simulink model "simulation_Hippocampus_compare_paper"  (R2023a)
settings: Solver=ode3  StartTime=0  StopTime=120  FixedStep=0.001  MaxStep=0.001  MinStep=0.00001  RelTol=1e-5  AbsTol=1e-5  EnableMultiTasking=on
values from neighbouring files (symbols this model uses):
  k_pos_ndi = 8    [parameters.m]
  k_vel_ndi = 8    [parameters.m]
  Kf = 6    [parameters.m]
  Kp = 0.01    [parameters.m]
  Kp_p = 30    [parameters.m]
  Kp_pitch = 8    [parameters.m]
  Kp_q = 10    [parameters.m]
  Kp_r = 10    [parameters.m]
  Kp_roll = 10    [parameters.m]
  Kp_u = 8    [parameters.m]
  Kp_yaw = 8    [parameters.m]
  Kq = 5    [parameters.m]
  Kr = 8    [parameters.m]
  Ktau1 = 0.1    [parameters.m]
  Ktau2 = 5    [parameters.m]
  Ktau3 = 5    [parameters.m]
  Ku = 8    [parameters.m]
  p11 = 0.4    [parameters.m]
  p12 = 0.2    [parameters.m]
  p21 = 0.2    [parameters.m]
  p22 = 0.05    [parameters.m]
  p31 = 0.3    [parameters.m]
  p32 = 0.05    [parameters.m]
  p41 = 0.5    [parameters.m]
  p42 = 0.1    [parameters.m]
  p51 = 0.5    [parameters.m]
  p52 = 0.1    [parameters.m]
  p61 = 0.5    [parameters.m]
  p62 = 0.1    [parameters.m]
  Q1 = -8    [simulation_para.m]
  Q2 = -10    [simulation_para.m]
  Q3 = -[0.01,5,8]    [simulation_para.m]
  Q4 = -[0.001,0.1,0.1]    [simulation_para.m]
  r1 = 4    [parameters.m]
  r2 = 6    [parameters.m]
libraries: simulink x8
(part 3 of 7)

== system simulation_Hippocampus_compare_paper/Proposed Linear gain/Disturbance: All derivatives2/disturbance3 ==
  note: Subsystem
  a : Inport
  a1 : Inport  Port=2
  Constant : Constant  Value=10
  Constant2 : Constant  Value=10
  Constant3 : Constant  Value=45
  Constant4 : Constant  Value=20
  Gain : Gain  Gain=pi/180
  Gain1 : Gain  Gain=pi/180
  MATLAB Function : MATLAB Function  TreatAsAtomicUnit=on
  Mux : Mux  Inputs=3
  Subsystem1 : Subsystem
  d : Outport
  wires:
  Subsystem1/1(Out1) -> MATLAB Function/3(u_wave)
  Constant/1 -> MATLAB Function/5(u_un)
  Mux/1 -> MATLAB Function/4(u_c)
  MATLAB Function/1(d) -> d/1
  a1/1 -> MATLAB Function/1(p)
  a/1 -> MATLAB Function/2(a)
  Constant4/1 -> Mux/1
  Gain/1 -> Mux/2
  Gain1/1 -> Mux/3
  Constant3/1 -> Gain1/1
  Constant2/1 -> Gain/1

== system simulation_Hippocampus_compare_paper/Proposed Linear gain/Disturbance: All derivatives2/old disturbance ==
  Gain : Gain  Gain=ones(12,1)  Multiplication=Matrix(K*u)
  Step : Step  Time=50  After=0.5  SampleTime=0
  Step1 : Step  Time=55  After=-0.5  SampleTime=0
  Step2 : Step  Time=100  After=0.5  SampleTime=0
  Step3 : Step  Time=105  After=-0.5  SampleTime=0
  Sum : Sum  Inputs=|++
  Sum2 : Sum  Inputs=|++
  Sum3 : Sum  Inputs=|++
  Out1 : Outport
  wires:
  Gain/1 -> Out1/1
  Sum3/1 -> Gain/1
  Step3/1 -> Sum2/2
  Step/1 -> Sum/1
  Step1/1 -> Sum/2
  Step2/1 -> Sum2/1
  Sum/1 -> Sum3/1
  Sum2/1 -> Sum3/2

== system simulation_Hippocampus_compare_paper/Proposed Linear gain/HippCampus/Subsystem ==
  In1 : Inport
  Demux : Demux  Outputs=[5 1 1 1 4]
  MATLAB Function : MATLAB Function  TreatAsAtomicUnit=on
  Mux : Mux  Inputs=5
  state : Outport
  wires:
  Demux/2 -> MATLAB Function/1(u)
  MATLAB Function/1(y) -> Mux/2
  In1/1 -> Demux/1
  Demux/3 -> Mux/3
  Demux/1 -> Mux/1
  Mux/1 -> state/1
  Demux/5 -> Mux/5
  Demux/4 -> Mux/4

== system simulation_Hippocampus_compare_paper/Proposed Linear gain/HippCampus/Subsystem1 ==
  u : Inport
  Integrator2 : Integrator
  Sqrt1 : Sqrt
  norm1 : MATLAB Function  TreatAsAtomicUnit=on
  Out1 : Outport
  wires:
  norm1/1(y) -> Integrator2/1
  Sqrt1/1 -> Out1/1
  Integrator2/1 -> Sqrt1/1
  u/1 -> norm1/1(u)

== system simulation_Hippocampus_compare_paper/Proposed Linear gain/HippCampus/Subsystem4 ==
  u : Inport
  Demux : Demux
  Mux : Mux
  Subsystem : Subsystem
  Subsystem1 : Subsystem
  Subsystem2 : Subsystem
  Subsystem3 : Subsystem
  Out1 : Outport
  wires:
  Subsystem2/1(Out1) -> Mux/3
  Demux/4 -> Subsystem3/1(u)
  Demux/3 -> Subsystem2/1(u)
  Subsystem1/1(Out1) -> Mux/2
  Demux/2 -> Subsystem1/1(u)
  Subsystem3/1(Out1) -> Mux/4
  Demux/1 -> Subsystem/1(u)
  Subsystem/1(Out1) -> Mux/1
  Mux/1 -> Out1/1
  u/1 -> Demux/1

== system simulation_Hippocampus_compare_paper/Proposed Linear gain1/Controller/calculate derivative 1 ==
  In1 : Inport
  Clock : Clock
  Derivative : Derivative
  MATLAB Function : MATLAB Function  TreatAsAtomicUnit=on
  Saturation : Saturate  UpperLimit=[6;3;6;6]  LowerLimit=-[6;3;6;6]
  y : Outport
  wires:
  Clock/1 -> MATLAB Function/2(t)
  In1/1 -> Derivative/1
  MATLAB Function/1(y) -> Saturation/1
  Derivative/1 -> MATLAB Function/1(u)
  Saturation/1 -> y/1

== system simulation_Hippocampus_compare_paper/Proposed Linear gain1/Disturbance: All derivatives1/disturbance2 ==
  Gain : Gain  Gain=[0;0;0;0;0;0;1;1;1;1;1;1]  Multiplication=Matrix(K*u)
  Step2 : Step  Time=60  After=0.5  SampleTime=0
  Step3 : Step  Time=55  After=0  SampleTime=0
  Sum1 : Sum
  Out1 : Outport
  wires:
  Step2/1 -> Sum1/1
  Step3/1 -> Sum1/2
  Gain/1 -> Out1/1
  Sum1/1 -> Gain/1

== system simulation_Hippocampus_compare_paper/Proposed Linear gain1/Disturbance: All derivatives1/disturbance3 ==
  note: Subsystem
  a : Inport
  a1 : Inport  Port=2
  Constant : Constant  Value=10
  Constant2 : Constant  Value=10
  Constant3 : Constant  Value=45
  Constant4 : Constant  Value=20
  Gain : Gain  Gain=pi/180
  Gain1 : Gain  Gain=pi/180
  MATLAB Function : MATLAB Function  TreatAsAtomicUnit=on
  Mux : Mux  Inputs=3
  Subsystem1 : Subsystem
  d : Outport
  wires:
  Subsystem1/1(Out1) -> MATLAB Function/3(u_wave)
  Constant/1 -> MATLAB Function/5(u_un)
  Mux/1 -> MATLAB Function/4(u_c)
  MATLAB Function/1(d) -> d/1
  a1/1 -> MATLAB Function/1(p)
  a/1 -> MATLAB Function/2(a)
  Constant4/1 -> Mux/1
  Gain/1 -> Mux/2
  Gain1/1 -> Mux/3
  Constant3/1 -> Gain1/1
  Constant2/1 -> Gain/1

== system simulation_Hippocampus_compare_paper/Proposed Linear gain1/Disturbance: All derivatives1/old disturbance ==
  Gain : Gain  Gain=ones(12,1)  Multiplication=Matrix(K*u)
  Step : Step  Time=50  After=0.5  SampleTime=0
  Step1 : Step  Time=55  After=-0.5  SampleTime=0
  Step2 : Step  Time=100  After=0.5  SampleTime=0
  Step3 : Step  Time=105  After=-0.5  SampleTime=0
  Sum : Sum  Inputs=|++
  Sum2 : Sum  Inputs=|++
  Sum3 : Sum  Inputs=|++
  Out1 : Outport
  wires:
  Gain/1 -> Out1/1
  Sum3/1 -> Gain/1
  Step3/1 -> Sum2/2
  Step/1 -> Sum/1
  Step1/1 -> Sum/2
  Step2/1 -> Sum2/1
  Sum/1 -> Sum3/1
  Sum2/1 -> Sum3/2

== system simulation_Hippocampus_compare_paper/Proposed Linear gain1/HippCampus/Subsystem ==
  In1 : Inport
  Demux : Demux  Outputs=[5 1 1 1 4]
  MATLAB Function : MATLAB Function  TreatAsAtomicUnit=on
  Mux : Mux  Inputs=5
  state : Outport
  wires:
  Demux/2 -> MATLAB Function/1(u)
  MATLAB Function/1(y) -> Mux/2
  In1/1 -> Demux/1
  Demux/3 -> Mux/3
  Demux/1 -> Mux/1
  Mux/1 -> state/1
  Demux/5 -> Mux/5
  Demux/4 -> Mux/4

== system simulation_Hippocampus_compare_paper/Proposed Linear gain1/HippCampus/Subsystem1 ==
  u : Inport
  Integrator2 : Integrator
  Sqrt1 : Sqrt
  norm1 : MATLAB Function  TreatAsAtomicUnit=on
  Out1 : Outport
  wires:
  norm1/1(y) -> Integrator2/1
  Sqrt1/1 -> Out1/1
  Integrator2/1 -> Sqrt1/1
  u/1 -> norm1/1(u)

== system simulation_Hippocampus_compare_paper/Proposed Linear gain1/HippCampus/Subsystem4 ==
  u : Inport
  Demux : Demux
  Mux : Mux
  Subsystem : Subsystem
  Subsystem1 : Subsystem
  Subsystem2 : Subsystem
  Subsystem3 : Subsystem
  Out1 : Outport
  wires:
  Subsystem2/1(Out1) -> Mux/3
  Demux/4 -> Subsystem3/1(u)
  Demux/3 -> Subsystem2/1(u)
  Subsystem1/1(Out1) -> Mux/2
  Demux/2 -> Subsystem1/1(u)
  Subsystem3/1(Out1) -> Mux/4
  Demux/1 -> Subsystem/1(u)
  Subsystem/1(Out1) -> Mux/1
  Mux/1 -> Out1/1
  u/1 -> Demux/1

== system simulation_Hippocampus_compare_paper/Proposed nonlinear gain/Controller/calculate derivative 1 ==
  In1 : Inport
  Clock : Clock
  Derivative : Derivative
  MATLAB Function : MATLAB Function  TreatAsAtomicUnit=on
  Saturation : Saturate  UpperLimit=[6;3;6;6]  LowerLimit=-[6;3;6;6]
  y : Outport
  wires:
  Clock/1 -> MATLAB Function/2(t)
  In1/1 -> Derivative/1
  MATLAB Function/1(y) -> Saturation/1
  Derivative/1 -> MATLAB Function/1(u)
  Saturation/1 -> y/1

== system simulation_Hippocampus_compare_paper/Proposed nonlinear gain/Disturbance: All derivatives1/disturbance2 ==
  Gain : Gain  Gain=[0;0;0;0;0;0;1;1;1;1;1;1]  Multiplication=Matrix(K*u)
  Step2 : Step  Time=60  After=0.5  SampleTime=0
  Step3 : Step  Time=55  After=0  SampleTime=0
  Sum1 : Sum
  Out1 : Outport
  wires:
  Step2/1 -> Sum1/1
  Step3/1 -> Sum1/2
  Gain/1 -> Out1/1
  Sum1/1 -> Gain/1

== system simulation_Hippocampus_compare_paper/Proposed nonlinear gain/Disturbance: All derivatives1/disturbance3 ==
  note: Subsystem
  a : Inport
  a1 : Inport  Port=2
  Constant : Constant  Value=10
  Constant2 : Constant  Value=10
  Constant3 : Constant  Value=45
  Constant4 : Constant  Value=20
  Gain : Gain  Gain=pi/180
  Gain1 : Gain  Gain=pi/180
  MATLAB Function : MATLAB Function  TreatAsAtomicUnit=on
  Mux : Mux  Inputs=3
  Subsystem1 : Subsystem
  d : Outport
  wires:
  Subsystem1/1(Out1) -> MATLAB Function/3(u_wave)
  Constant/1 -> MATLAB Function/5(u_un)
  Mux/1 -> MATLAB Function/4(u_c)
  MATLAB Function/1(d) -> d/1
  a1/1 -> MATLAB Function/1(p)
  a/1 -> MATLAB Function/2(a)
  Constant4/1 -> Mux/1
  Gain/1 -> Mux/2
  Gain1/1 -> Mux/3
  Constant3/1 -> Gain1/1
  Constant2/1 -> Gain/1

== system simulation_Hippocampus_compare_paper/Proposed nonlinear gain/Disturbance: All derivatives1/old disturbance ==
  Gain : Gain  Gain=ones(12,1)  Multiplication=Matrix(K*u)
  Step : Step  Time=50  After=0.5  SampleTime=0
  Step1 : Step  Time=55  After=-0.5  SampleTime=0
  Step2 : Step  Time=100  After=0.5  SampleTime=0
  Step3 : Step  Time=105  After=-0.5  SampleTime=0
  Sum : Sum  Inputs=|++
  Sum2 : Sum  Inputs=|++
  Sum3 : Sum  Inputs=|++
  Out1 : Outport
  wires:
  Gain/1 -> Out1/1
  Sum3/1 -> Gain/1
  Step3/1 -> Sum2/2
  Step/1 -> Sum/1
  Step1/1 -> Sum/2
  Step2/1 -> Sum2/1
  Sum/1 -> Sum3/1
  Sum2/1 -> Sum3/2

== system simulation_Hippocampus_compare_paper/Proposed nonlinear gain/HippCampus/Subsystem ==
  In1 : Inport
  Demux : Demux  Outputs=[5 1 1 1 4]
  MATLAB Function : MATLAB Function  TreatAsAtomicUnit=on
  Mux : Mux  Inputs=5
  state : Outport
  wires:
  Demux/2 -> MATLAB Function/1(u)
  MATLAB Function/1(y) -> Mux/2
  In1/1 -> Demux/1
  Demux/3 -> Mux/3
  Demux/1 -> Mux/1
  Mux/1 -> state/1
  Demux/5 -> Mux/5
  Demux/4 -> Mux/4

== system simulation_Hippocampus_compare_paper/Proposed nonlinear gain/HippCampus/Subsystem1 ==
  u : Inport
  Integrator2 : Integrator
  Sqrt1 : Sqrt
  norm1 : MATLAB Function  TreatAsAtomicUnit=on
  Out1 : Outport
  wires:
  norm1/1(y) -> Integrator2/1
  Sqrt1/1 -> Out1/1
  Integrator2/1 -> Sqrt1/1
  u/1 -> norm1/1(u)

== system simulation_Hippocampus_compare_paper/Proposed nonlinear gain/HippCampus/Subsystem4 ==
  u : Inport
  Demux : Demux
  Mux : Mux
  Subsystem : Subsystem
  Subsystem1 : Subsystem
  Subsystem2 : Subsystem
  Subsystem3 : Subsystem
  Out1 : Outport
  wires:
  Subsystem2/1(Out1) -> Mux/3
  Demux/4 -> Subsystem3/1(u)
  Demux/3 -> Subsystem2/1(u)
  Subsystem1/1(Out1) -> Mux/2
  Demux/2 -> Subsystem1/1(u)
  Subsystem3/1(Out1) -> Mux/4
  Demux/1 -> Subsystem/1(u)
  Subsystem/1(Out1) -> Mux/1
  Mux/1 -> Out1/1
  u/1 -> Demux/1

== system simulation_Hippocampus_compare_paper/Proposed nonlinear gain1/Controller/calculate derivative 1 ==
  In1 : Inport
  Clock : Clock
  Derivative : Derivative
  MATLAB Function : MATLAB Function  TreatAsAtomicUnit=on
  Saturation : Saturate  UpperLimit=[6;3;6;6]  LowerLimit=-[6;3;6;6]
  y : Outport
  wires:
  Clock/1 -> MATLAB Function/2(t)
  In1/1 -> Derivative/1
  MATLAB Function/1(y) -> Saturation/1
  Derivative/1 -> MATLAB Function/1(u)
  Saturation/1 -> y/1

== system simulation_Hippocampus_compare_paper/Proposed nonlinear gain1/Disturbance: All derivatives1/disturbance2 ==
  Gain : Gain  Gain=[0;0;0;0;0;0;1;1;1;1;1;1]  Multiplication=Matrix(K*u)
  Step2 : Step  Time=60  After=0.5  SampleTime=0
  Step3 : Step  Time=55  After=0  SampleTime=0
  Sum1 : Sum
  Out1 : Outport
  wires:
  Step2/1 -> Sum1/1
  Step3/1 -> Sum1/2
  Gain/1 -> Out1/1
  Sum1/1 -> Gain/1

== system simulation_Hippocampus_compare_paper/Proposed nonlinear gain1/Disturbance: All derivatives1/disturbance3 ==
  note: Subsystem
  a : Inport
  a1 : Inport  Port=2
  Constant : Constant  Value=10
  Constant2 : Constant  Value=10
  Constant3 : Constant  Value=45
  Constant4 : Constant  Value=20
  Gain : Gain  Gain=pi/180
  Gain1 : Gain  Gain=pi/180
  MATLAB Function : MATLAB Function  TreatAsAtomicUnit=on
  Mux : Mux  Inputs=3
  Subsystem1 : Subsystem
  d : Outport
  wires:
  Subsystem1/1(Out1) -> MATLAB Function/3(u_wave)
  Constant/1 -> MATLAB Function/5(u_un)
  Mux/1 -> MATLAB Function/4(u_c)
  MATLAB Function/1(d) -> d/1
  a1/1 -> MATLAB Function/1(p)
  a/1 -> MATLAB Function/2(a)
  Constant4/1 -> Mux/1
  Gain/1 -> Mux/2
  Gain1/1 -> Mux/3
  Constant3/1 -> Gain1/1
  Constant2/1 -> Gain/1

== system simulation_Hippocampus_compare_paper/Proposed nonlinear gain1/Disturbance: All derivatives1/old disturbance ==
  Gain : Gain  Gain=ones(12,1)  Multiplication=Matrix(K*u)
  Step : Step  Time=50  After=0.5  SampleTime=0
  Step1 : Step  Time=55  After=-0.5  SampleTime=0
  Step2 : Step  Time=100  After=0.5  SampleTime=0
  Step3 : Step  Time=105  After=-0.5  SampleTime=0
  Sum : Sum  Inputs=|++
  Sum2 : Sum  Inputs=|++
  Sum3 : Sum  Inputs=|++
  Out1 : Outport
  wires:
  Gain/1 -> Out1/1
  Sum3/1 -> Gain/1
  Step3/1 -> Sum2/2
  Step/1 -> Sum/1
  Step1/1 -> Sum/2
  Step2/1 -> Sum2/1
  Sum/1 -> Sum3/1
  Sum2/1 -> Sum3/2

== system simulation_Hippocampus_compare_paper/Proposed nonlinear gain1/HippCampus/Subsystem ==
  In1 : Inport
  Demux : Demux  Outputs=[5 1 1 1 4]
  MATLAB Function : MATLAB Function  TreatAsAtomicUnit=on
  Mux : Mux  Inputs=5
  state : Outport
  wires:
  Demux/2 -> MATLAB Function/1(u)
  MATLAB Function/1(y) -> Mux/2
  In1/1 -> Demux/1
  Demux/3 -> Mux/3
  Demux/1 -> Mux/1
  Mux/1 -> state/1
  Demux/5 -> Mux/5
  Demux/4 -> Mux/4

== system simulation_Hippocampus_compare_paper/Proposed nonlinear gain1/HippCampus/Subsystem1 ==
  u : Inport
  Integrator2 : Integrator
  Sqrt1 : Sqrt
  norm1 : MATLAB Function  TreatAsAtomicUnit=on
  Out1 : Outport
  wires:
  norm1/1(y) -> Integrator2/1
  Sqrt1/1 -> Out1/1
  Integrator2/1 -> Sqrt1/1
  u/1 -> norm1/1(u)

== system simulation_Hippocampus_compare_paper/Proposed nonlinear gain1/HippCampus/Subsystem4 ==
  u : Inport
  Demux : Demux
  Mux : Mux
  Subsystem : Subsystem
  Subsystem1 : Subsystem
  Subsystem2 : Subsystem
  Subsystem3 : Subsystem
  Out1 : Outport
  wires:
  Subsystem2/1(Out1) -> Mux/3
  Demux/4 -> Subsystem3/1(u)
  Demux/3 -> Subsystem2/1(u)
  Subsystem1/1(Out1) -> Mux/2
  Demux/2 -> Subsystem1/1(u)
  Subsystem3/1(Out1) -> Mux/4
  Demux/1 -> Subsystem/1(u)
  Subsystem/1(Out1) -> Mux/1
  Mux/1 -> Out1/1
  u/1 -> Demux/1

== system simulation_Hippocampus_compare_paper/Proposed nonlinear gain2/Controller/calculate derivative 1 ==
  In1 : Inport
  Clock : Clock
  Derivative : Derivative
  MATLAB Function : MATLAB Function  TreatAsAtomicUnit=on
  Saturation : Saturate  UpperLimit=[6;3;6;6]  LowerLimit=-[6;3;6;6]
  y : Outport
  wires:
  Clock/1 -> MATLAB Function/2(t)
  In1/1 -> Derivative/1
  MATLAB Function/1(y) -> Saturation/1
  Derivative/1 -> MATLAB Function/1(u)
  Saturation/1 -> y/1

== system simulation_Hippocampus_compare_paper/Proposed nonlinear gain2/HippCampus/Subsystem ==
  In1 : Inport
  Demux : Demux  Outputs=[5 1 1 1 4]
  MATLAB Function : MATLAB Function  TreatAsAtomicUnit=on
  Mux : Mux  Inputs=5
  state : Outport
  wires:
  Demux/2 -> MATLAB Function/1(u)
  MATLAB Function/1(y) -> Mux/2
  In1/1 -> Demux/1
  Demux/3 -> Mux/3
  Demux/1 -> Mux/1
  Mux/1 -> state/1
  Demux/5 -> Mux/5
  Demux/4 -> Mux/4

== system simulation_Hippocampus_compare_paper/Proposed nonlinear gain2/HippCampus/Subsystem1 ==
  u : Inport
  Integrator2 : Integrator
  Sqrt1 : Sqrt
  norm1 : MATLAB Function  TreatAsAtomicUnit=on
  Out1 : Outport
  wires:
  norm1/1(y) -> Integrator2/1
  Sqrt1/1 -> Out1/1
  Integrator2/1 -> Sqrt1/1
  u/1 -> norm1/1(u)

== system simulation_Hippocampus_compare_paper/Proposed nonlinear gain2/HippCampus/Subsystem4 ==
  u : Inport
  Demux : Demux
  Mux : Mux
  Subsystem : Subsystem
  Subsystem1 : Subsystem
  Subsystem2 : Subsystem
  Subsystem3 : Subsystem
  Out1 : Outport
  wires:
  Subsystem2/1(Out1) -> Mux/3
  Demux/4 -> Subsystem3/1(u)
  Demux/3 -> Subsystem2/1(u)
  Subsystem1/1(Out1) -> Mux/2
  Demux/2 -> Subsystem1/1(u)
  Subsystem3/1(Out1) -> Mux/4
  Demux/1 -> Subsystem/1(u)
  Subsystem/1(Out1) -> Mux/1
  Mux/1 -> Out1/1
  u/1 -> Demux/1

== system simulation_Hippocampus_compare_paper/Stabilizing without v w /Controller/calculate derivative 1 ==
  In1 : Inport
  Clock : Clock
  Derivative : Derivative
  MATLAB Function : MATLAB Function  TreatAsAtomicUnit=on
  Saturation : Saturate  UpperLimit=[6;3;6;6]  LowerLimit=-[6;3;6;6]
  y : Outport
  wires:
  Clock/1 -> MATLAB Function/2(t)
  In1/1 -> Derivative/1
  MATLAB Function/1(y) -> Saturation/1
  Derivative/1 -> MATLAB Function/1(u)
  Saturation/1 -> y/1

== system simulation_Hippocampus_compare_paper/Stabilizing without v w /HippCampus/Subsystem ==
  In1 : Inport
  Demux : Demux  Outputs=[5 1 1 1 4]
  MATLAB Function : MATLAB Function  TreatAsAtomicUnit=on
  Mux : Mux  Inputs=5
  state : Outport
  wires:
  Demux/2 -> MATLAB Function/1(u)
  MATLAB Function/1(y) -> Mux/2
  In1/1 -> Demux/1
  Demux/3 -> Mux/3
  Demux/1 -> Mux/1
  Mux/1 -> state/1
  Demux/5 -> Mux/5
  Demux/4 -> Mux/4

== system simulation_Hippocampus_compare_paper/Stabilizing without v w /HippCampus/Subsystem1 ==
  u : Inport
  Integrator2 : Integrator
  Sqrt1 : Sqrt
  norm1 : MATLAB Function  TreatAsAtomicUnit=on
  Out1 : Outport
  wires:
  norm1/1(y) -> Integrator2/1
  Sqrt1/1 -> Out1/1
  Integrator2/1 -> Sqrt1/1
  u/1 -> norm1/1(u)

== system simulation_Hippocampus_compare_paper/Stabilizing without v w /HippCampus/Subsystem4 ==
  u : Inport
  Demux : Demux
  Mux : Mux
  Subsystem : Subsystem
  Subsystem1 : Subsystem
  Subsystem2 : Subsystem
  Subsystem3 : Subsystem
  Out1 : Outport
  wires:
  Subsystem2/1(Out1) -> Mux/3
  Demux/4 -> Subsystem3/1(u)
  Demux/3 -> Subsystem2/1(u)
  Subsystem1/1(Out1) -> Mux/2
  Demux/2 -> Subsystem1/1(u)
  Subsystem3/1(Out1) -> Mux/4
  Demux/1 -> Subsystem/1(u)
  Subsystem/1(Out1) -> Mux/1
  Mux/1 -> Out1/1
  u/1 -> Demux/1

== system simulation_Hippocampus_compare_paper/Stabilizing without v w 1/Controller/calculate derivative  ==
  In1 : Inport
  Clock : Clock
  Derivative : Derivative
  MATLAB Function : MATLAB Function  TreatAsAtomicUnit=on
  Saturation : Saturate  UpperLimit=[10;10;10;10]  LowerLimit=-[10;10;10;10]
  y : Outport
  wires:
  Clock/1 -> MATLAB Function/2(t)
  In1/1 -> Derivative/1
  MATLAB Function/1(y) -> Saturation/1
  Derivative/1 -> MATLAB Function/1(u)
  Saturation/1 -> y/1

== system simulation_Hippocampus_compare_paper/Stabilizing without v w 1/HippCampus/Subsystem ==
  In1 : Inport
  Demux : Demux  Outputs=[5 1 1 1 4]
  MATLAB Function : MATLAB Function  TreatAsAtomicUnit=on
  Mux : Mux  Inputs=5
  state : Outport
  wires:
  Demux/2 -> MATLAB Function/1(u)
  MATLAB Function/1(y) -> Mux/2
  In1/1 -> Demux/1
  Demux/3 -> Mux/3
  Demux/1 -> Mux/1
  Mux/1 -> state/1
  Demux/5 -> Mux/5
  Demux/4 -> Mux/4

== system simulation_Hippocampus_compare_paper/Stabilizing without v w 1/HippCampus/Subsystem1 ==
  u : Inport
  Integrator2 : Integrator
  Sqrt1 : Sqrt
  norm1 : MATLAB Function  TreatAsAtomicUnit=on
  Out1 : Outport
  wires:
  norm1/1(y) -> Integrator2/1
  Sqrt1/1 -> Out1/1
  Integrator2/1 -> Sqrt1/1
  u/1 -> norm1/1(u)

== system simulation_Hippocampus_compare_paper/Stabilizing without v w 1/HippCampus/Subsystem4 ==
  u : Inport
  Demux : Demux
  Mux : Mux
  Subsystem : Subsystem
  Subsystem1 : Subsystem
  Subsystem2 : Subsystem
  Subsystem3 : Subsystem
  Out1 : Outport
  wires:
  Subsystem2/1(Out1) -> Mux/3
  Demux/4 -> Subsystem3/1(u)
  Demux/3 -> Subsystem2/1(u)
  Subsystem1/1(Out1) -> Mux/2
  Demux/2 -> Subsystem1/1(u)
  Subsystem3/1(Out1) -> Mux/4
  Demux/1 -> Subsystem/1(u)
  Subsystem/1(Out1) -> Mux/1
  Mux/1 -> Out1/1
  u/1 -> Demux/1

== system simulation_Hippocampus_compare_paper/NDI/Controller/Subsystem/Subsystem1 ==
  rpy_ref : Inport
  state : Inport  Port=2
  Add1 : Sum  Inputs=+-
  Add2 : Sum  Inputs=+-
  Add3 : Sum  Inputs=+-
  Demux1 : Demux  Outputs=3
  Demux2 : Demux  Outputs=3
  Gain : Gain  Gain=Kp_roll
  Gain1 : Gain  Gain=Kp_yaw
  Gain2 : Gain  Gain=Kp_pitch
  Mux2 : Mux  Inputs=3
  Subsystem : Subsystem
  pqr_ref : Outport
  wires:
  state/1 -> Subsystem/1(x)
  Demux1/1 -> Add1/2
  Demux1/3 -> Add3/2
  Demux2/3 -> Add3/1
  Demux1/2 -> Add2/2
  Gain/1 -> Mux2/1
  Gain1/1 -> Mux2/3
  Add2/1 -> Gain2/1
  Gain2/1 -> Mux2/2
  Demux2/2 -> Add2/1
  Demux2/1 -> Add1/1
  Subsystem/1(rpy) -> Demux1/1
  rpy_ref/1 -> Demux2/1
  Add1/1 -> Gain/1
  Add3/1 -> Gain1/1
  Mux2/1 -> pqr_ref/1

== system simulation_Hippocampus_compare_paper/NDI/Controller/Subsystem/Subsystem2 ==
  state : Inport
  upqr_ref : Inport  Port=2
  Add{,1..4} (5 alike) : Sum  Inputs=+-
  Demux : Demux
  Demux1 : Demux
  Divide : Product  Inputs=**  Multiplication=Matrix(*)
  Gain : Gain  Gain=Kp_p
  Gain1 : Gain  Gain=Kp_r
  Gain2 : Gain  Gain=Kp_q
  Gain3 : Gain  Gain=Kp_u
  Mux : Mux
  NDI : Subsystem
  Subsystem : Subsystem
  tau : Outport
  wires:
  Add1/1 -> Gain/1
  NDI/1(Lg_h_inv) -> Divide/1
  Mux/1 -> Add/1
  Add2/1 -> Gain2/1
  Add3/1 -> Gain1/1
  Divide/1 -> tau/1
  NDI/2(Lf_h) -> Add/2
  Add/1 -> Divide/2
  state/1 -> Subsystem/1(x), NDI/1(state)
  Subsystem/1(upqr) -> Demux/1
  Demux1/2 -> Add1/1
  Demux1/3 -> Add2/1
  Demux1/4 -> Add3/1
  upqr_ref/1 -> Demux1/1
  Gain1/1 -> Mux/4
  Gain2/1 -> Mux/3
  Gain/1 -> Mux/2
  Add4/1 -> Gain3/1
  Gain3/1 -> Mux/1
  Demux/1 -> Add4/2
  Demux/2 -> Add1/2
  Demux/3 -> Add2/2
  Demux/4 -> Add3/2
  Demux1/1 -> Add4/1

== system simulation_Hippocampus_compare_paper/NDI/Disturbance: All derivatives1/disturbance3/Subsystem ==
  Constant2 : Constant  Value=5
  Constant3 : Constant  Value=30
  Constant4 : Constant  Value=20
  Gain : Gain  Gain=pi/180
  Gain1 : Gain  Gain=pi/180
  Mux : Mux  Inputs=3
  Out1 : Outport
  wires:
  Constant2/1 -> Gain/1
  Constant3/1 -> Gain1/1
  Gain1/1 -> Mux/3
  Gain/1 -> Mux/2
  Mux/1 -> Out1/1
  Constant4/1 -> Mux/1

== system simulation_Hippocampus_compare_paper/NDI/Disturbance: All derivatives1/disturbance3/Subsystem1 ==
  Clock : Clock
  Mux1 : Mux  Inputs=3
  wave frenquency : Subsystem
  wave percentage : Subsystem
  Out1 : Outport
  wires:
  wave frenquency/1(Out1) -> Mux1/2
  Mux1/1 -> Out1/1
  wave percentage/1(Out1) -> Mux1/1
  Clock/1 -> Mux1/3

== system simulation_Hippocampus_compare_paper/NDI/Disturbance: All derivatives2/disturbance3/Subsystem1 ==
  Clock : Clock
  Mux1 : Mux  Inputs=3
  wave frenquency : Subsystem
  wave percentage : Subsystem
  Out1 : Outport
  wires:
  wave frenquency/1(Out1) -> Mux1/2
  Mux1/1 -> Out1/1
  wave percentage/1(Out1) -> Mux1/1
  Clock/1 -> Mux1/3

== system simulation_Hippocampus_compare_paper/NDI/HippCampus1/Subsystem4/Subsystem ==
  u : Inport
  Integrator2 : Integrator
  Sqrt1 : Sqrt
  norm1 : MATLAB Function  TreatAsAtomicUnit=on
  Out1 : Outport
  wires:
  norm1/1(y) -> Integrator2/1
  Sqrt1/1 -> Out1/1
  Integrator2/1 -> Sqrt1/1
  u/1 -> norm1/1(u)

== system simulation_Hippocampus_compare_paper/NDI/HippCampus1/Subsystem4/Subsystem1 ==
  u : Inport
  Integrator2 : Integrator
  Sqrt1 : Sqrt
  norm1 : MATLAB Function  TreatAsAtomicUnit=on
  Out1 : Outport
  wires:
  norm1/1(y) -> Integrator2/1
  Sqrt1/1 -> Out1/1
  Integrator2/1 -> Sqrt1/1
  u/1 -> norm1/1(u)

== system simulation_Hippocampus_compare_paper/NDI/HippCampus1/Subsystem4/Subsystem2 ==
  u : Inport
  Integrator2 : Integrator
  Sqrt1 : Sqrt
  norm1 : MATLAB Function  TreatAsAtomicUnit=on
  Out1 : Outport
  wires:
  norm1/1(y) -> Integrator2/1
  Sqrt1/1 -> Out1/1
  Integrator2/1 -> Sqrt1/1
  u/1 -> norm1/1(u)

== system simulation_Hippocampus_compare_paper/NDI/HippCampus1/Subsystem4/Subsystem3 ==
  u : Inport
  Integrator2 : Integrator
  Sqrt1 : Sqrt
  norm1 : MATLAB Function  TreatAsAtomicUnit=on
  Out1 : Outport
  wires:
  norm1/1(y) -> Integrator2/1
  Sqrt1/1 -> Out1/1
  Integrator2/1 -> Sqrt1/1
  u/1 -> norm1/1(u)

== system simulation_Hippocampus_compare_paper/NDI4/Controller/Subsystem/Subsystem1 ==
  rpy_ref : Inport
  state : Inport  Port=2
  Add1 : Sum  Inputs=+-
  Add2 : Sum  Inputs=+-
  Add3 : Sum  Inputs=+-
  Demux1 : Demux  Outputs=3
  Demux2 : Demux  Outputs=3
  Gain : Gain  Gain=Kp_roll
  Gain1 : Gain  Gain=Kp_yaw
  Gain2 : Gain  Gain=Kp_pitch
  Mux2 : Mux  Inputs=3
  Subsystem : Subsystem
  pqr_ref : Outport
  wires:
  state/1 -> Subsystem/1(x)
  Demux1/1 -> Add1/2
  Demux1/3 -> Add3/2
  Demux2/3 -> Add3/1
  Demux1/2 -> Add2/2
  Gain/1 -> Mux2/1
  Gain1/1 -> Mux2/3
  Add2/1 -> Gain2/1
  Gain2/1 -> Mux2/2
  Demux2/2 -> Add2/1
  Demux2/1 -> Add1/1
  Subsystem/1(rpy) -> Demux1/1
  rpy_ref/1 -> Demux2/1
  Add1/1 -> Gain/1
  Add3/1 -> Gain1/1
  Mux2/1 -> pqr_ref/1

== system simulation_Hippocampus_compare_paper/NDI4/Controller/Subsystem/Subsystem2 ==
  state : Inport
  upqr_ref : Inport  Port=2
  Add{,1..4} (5 alike) : Sum  Inputs=+-
  Demux : Demux
  Demux1 : Demux
  Divide : Product  Inputs=**  Multiplication=Matrix(*)
  Gain : Gain  Gain=Kp_p
  Gain1 : Gain  Gain=Kp_r
  Gain2 : Gain  Gain=Kp_q
  Gain3 : Gain  Gain=Kp_u
  Mux : Mux
  NDI : Subsystem
  Subsystem : Subsystem
  tau : Outport
  wires:
  Add1/1 -> Gain/1
  NDI/1(Lg_h_inv) -> Divide/1
  Mux/1 -> Add/1
  Add2/1 -> Gain2/1
  Add3/1 -> Gain1/1
  Divide/1 -> tau/1
  NDI/2(Lf_h) -> Add/2
  Add/1 -> Divide/2
  state/1 -> Subsystem/1(x), NDI/1(state)
  Subsystem/1(upqr) -> Demux/1
  Demux1/2 -> Add1/1
  Demux1/3 -> Add2/1
  Demux1/4 -> Add3/1
  upqr_ref/1 -> Demux1/1
  Gain1/1 -> Mux/4
  Gain2/1 -> Mux/3
  Gain/1 -> Mux/2
  Add4/1 -> Gain3/1
  Gain3/1 -> Mux/1
  Demux/1 -> Add4/2
  Demux/2 -> Add1/2
  Demux/3 -> Add2/2
  Demux/4 -> Add3/2
  Demux1/1 -> Add4/1

== system simulation_Hippocampus_compare_paper/NDI4/Disturbance: All derivatives1/disturbance3/Subsystem ==
  Constant2 : Constant  Value=5
  Constant3 : Constant  Value=30
  Constant4 : Constant  Value=20
  Gain : Gain  Gain=pi/180
  Gain1 : Gain  Gain=pi/180
  Mux : Mux  Inputs=3
  Out1 : Outport
  wires:
  Constant2/1 -> Gain/1
  Constant3/1 -> Gain1/1
  Gain1/1 -> Mux/3
  Gain/1 -> Mux/2
  Mux/1 -> Out1/1
  Constant4/1 -> Mux/1

== system simulation_Hippocampus_compare_paper/NDI4/Disturbance: All derivatives1/disturbance3/Subsystem1 ==
  Clock : Clock
  Mux1 : Mux  Inputs=3
  wave frenquency : Subsystem
  wave percentage : Subsystem
  Out1 : Outport
  wires:
  wave frenquency/1(Out1) -> Mux1/2
  Mux1/1 -> Out1/1
  wave percentage/1(Out1) -> Mux1/1
  Clock/1 -> Mux1/3

== system simulation_Hippocampus_compare_paper/NDI4/Disturbance: All derivatives2/disturbance3/Subsystem1 ==
  Clock : Clock
  Mux1 : Mux  Inputs=3
  wave frenquency : Subsystem
  wave percentage : Subsystem
  Out1 : Outport
  wires:
  wave frenquency/1(Out1) -> Mux1/2
  Mux1/1 -> Out1/1
  wave percentage/1(Out1) -> Mux1/1
  Clock/1 -> Mux1/3

== system simulation_Hippocampus_compare_paper/NDI4/HippCampus1/Subsystem4/Subsystem ==
  u : Inport
  Integrator2 : Integrator
  Sqrt1 : Sqrt
  norm1 : MATLAB Function  TreatAsAtomicUnit=on
  Out1 : Outport
  wires:
  norm1/1(y) -> Integrator2/1
  Sqrt1/1 -> Out1/1
  Integrator2/1 -> Sqrt1/1
  u/1 -> norm1/1(u)

== system simulation_Hippocampus_compare_paper/NDI4/HippCampus1/Subsystem4/Subsystem1 ==
  u : Inport
  Integrator2 : Integrator
  Sqrt1 : Sqrt
  norm1 : MATLAB Function  TreatAsAtomicUnit=on
  Out1 : Outport
  wires:
  norm1/1(y) -> Integrator2/1
  Sqrt1/1 -> Out1/1
  Integrator2/1 -> Sqrt1/1
  u/1 -> norm1/1(u)

== system simulation_Hippocampus_compare_paper/NDI4/HippCampus1/Subsystem4/Subsystem2 ==
  u : Inport
  Integrator2 : Integrator
  Sqrt1 : Sqrt
  norm1 : MATLAB Function  TreatAsAtomicUnit=on
  Out1 : Outport
  wires:
  norm1/1(y) -> Integrator2/1
  Sqrt1/1 -> Out1/1
  Integrator2/1 -> Sqrt1/1
  u/1 -> norm1/1(u)

== system simulation_Hippocampus_compare_paper/NDI4/HippCampus1/Subsystem4/Subsystem3 ==
  u : Inport
  Integrator2 : Integrator
  Sqrt1 : Sqrt
  norm1 : MATLAB Function  TreatAsAtomicUnit=on
  Out1 : Outport
  wires:
  norm1/1(y) -> Integrator2/1
  Sqrt1/1 -> Out1/1
  Integrator2/1 -> Sqrt1/1
  u/1 -> norm1/1(u)

== system simulation_Hippocampus_compare_paper/PDPD/Disturbance: All derivatives1/disturbance3/Subsystem1 ==
  Clock : Clock
  Mux1 : Mux  Inputs=3
  wave frenquency : Subsystem
  wave percentage : Subsystem
  Out1 : Outport
  wires:
  wave frenquency/1(Out1) -> Mux1/2
  Mux1/1 -> Out1/1
  wave percentage/1(Out1) -> Mux1/1
  Clock/1 -> Mux1/3

== system simulation_Hippocampus_compare_paper/PDPD/HippCampus1/Subsystem4/Subsystem ==
  u : Inport
  Integrator2 : Integrator
  Sqrt1 : Sqrt
  norm1 : MATLAB Function  TreatAsAtomicUnit=on
  Out1 : Outport
  wires:
  norm1/1(y) -> Integrator2/1
  Sqrt1/1 -> Out1/1
  Integrator2/1 -> Sqrt1/1
  u/1 -> norm1/1(u)

== system simulation_Hippocampus_compare_paper/PDPD/HippCampus1/Subsystem4/Subsystem1 ==
  u : Inport
  Integrator2 : Integrator
  Sqrt1 : Sqrt
  norm1 : MATLAB Function  TreatAsAtomicUnit=on
  Out1 : Outport
  wires:
  norm1/1(y) -> Integrator2/1
  Sqrt1/1 -> Out1/1
  Integrator2/1 -> Sqrt1/1
  u/1 -> norm1/1(u)

== system simulation_Hippocampus_compare_paper/PDPD/HippCampus1/Subsystem4/Subsystem2 ==
  u : Inport
  Integrator2 : Integrator
  Sqrt1 : Sqrt
  norm1 : MATLAB Function  TreatAsAtomicUnit=on
  Out1 : Outport
  wires:
  norm1/1(y) -> Integrator2/1
  Sqrt1/1 -> Out1/1
  Integrator2/1 -> Sqrt1/1
  u/1 -> norm1/1(u)

== system simulation_Hippocampus_compare_paper/PDPD/HippCampus1/Subsystem4/Subsystem3 ==
  u : Inport
  Integrator2 : Integrator
  Sqrt1 : Sqrt
  norm1 : MATLAB Function  TreatAsAtomicUnit=on
  Out1 : Outport
  wires:
  norm1/1(y) -> Integrator2/1
  Sqrt1/1 -> Out1/1
  Integrator2/1 -> Sqrt1/1
  u/1 -> norm1/1(u)

== system simulation_Hippocampus_compare_paper/PDPD1/Disturbance: All derivatives1/disturbance3/Subsystem1 ==
  Clock : Clock
  Mux1 : Mux  Inputs=3
  wave frenquency : Subsystem
  wave percentage : Subsystem
  Out1 : Outport
  wires:
  wave frenquency/1(Out1) -> Mux1/2
  Mux1/1 -> Out1/1
  wave percentage/1(Out1) -> Mux1/1
  Clock/1 -> Mux1/3

== system simulation_Hippocampus_compare_paper/PDPD1/HippCampus1/Subsystem4/Subsystem ==
  u : Inport
  Integrator2 : Integrator
  Sqrt1 : Sqrt
  norm1 : MATLAB Function  TreatAsAtomicUnit=on
  Out1 : Outport
  wires:
  norm1/1(y) -> Integrator2/1
  Sqrt1/1 -> Out1/1
  Integrator2/1 -> Sqrt1/1
  u/1 -> norm1/1(u)

== system simulation_Hippocampus_compare_paper/PDPD1/HippCampus1/Subsystem4/Subsystem1 ==
  u : Inport
  Integrator2 : Integrator
  Sqrt1 : Sqrt
  norm1 : MATLAB Function  TreatAsAtomicUnit=on
  Out1 : Outport
  wires:
  norm1/1(y) -> Integrator2/1
  Sqrt1/1 -> Out1/1
  Integrator2/1 -> Sqrt1/1
  u/1 -> norm1/1(u)

== system simulation_Hippocampus_compare_paper/PDPD1/HippCampus1/Subsystem4/Subsystem2 ==
  u : Inport
  Integrator2 : Integrator
  Sqrt1 : Sqrt
  norm1 : MATLAB Function  TreatAsAtomicUnit=on
  Out1 : Outport
  wires:
  norm1/1(y) -> Integrator2/1
  Sqrt1/1 -> Out1/1
  Integrator2/1 -> Sqrt1/1
  u/1 -> norm1/1(u)

== system simulation_Hippocampus_compare_paper/PDPD1/HippCampus1/Subsystem4/Subsystem3 ==
  u : Inport
  Integrator2 : Integrator
  Sqrt1 : Sqrt
  norm1 : MATLAB Function  TreatAsAtomicUnit=on
  Out1 : Outport
  wires:
  norm1/1(y) -> Integrator2/1
  Sqrt1/1 -> Out1/1
  Integrator2/1 -> Sqrt1/1
  u/1 -> norm1/1(u)

== system simulation_Hippocampus_compare_paper/Proposed Linear gain/Disturbance: All derivatives1/disturbance3/Subsystem1 ==
  Clock : Clock
  Mux1 : Mux  Inputs=3
  wave frenquency : Subsystem
  wave percentage : Subsystem
  Out1 : Outport
  wires:
  wave frenquency/1(Out1) -> Mux1/2
  Mux1/1 -> Out1/1
  wave percentage/1(Out1) -> Mux1/1
  Clock/1 -> Mux1/3

== system simulation_Hippocampus_compare_paper/Proposed Linear gain/Disturbance: All derivatives2/disturbance3/Subsystem1 ==
  Clock : Clock
  Mux1 : Mux  Inputs=3
  wave frenquency : Subsystem
  wave percentage : Subsystem
  Out1 : Outport
  wires:
  wave frenquency/1(Out1) -> Mux1/2
  Mux1/1 -> Out1/1
  wave percentage/1(Out1) -> Mux1/1
  Clock/1 -> Mux1/3

== system simulation_Hippocampus_compare_paper/Proposed Linear gain/HippCampus/Subsystem4/Subsystem ==
  u : Inport
  Integrator2 : Integrator
  Sqrt1 : Sqrt
  norm1 : MATLAB Function  TreatAsAtomicUnit=on
  Out1 : Outport
  wires:
  norm1/1(y) -> Integrator2/1
  Sqrt1/1 -> Out1/1
  Integrator2/1 -> Sqrt1/1
  u/1 -> norm1/1(u)

== system simulation_Hippocampus_compare_paper/Proposed Linear gain/HippCampus/Subsystem4/Subsystem1 ==
  u : Inport
  Integrator2 : Integrator
  Sqrt1 : Sqrt
  norm1 : MATLAB Function  TreatAsAtomicUnit=on
  Out1 : Outport
  wires:
  norm1/1(y) -> Integrator2/1
  Sqrt1/1 -> Out1/1
  Integrator2/1 -> Sqrt1/1
  u/1 -> norm1/1(u)

== system simulation_Hippocampus_compare_paper/Proposed Linear gain/HippCampus/Subsystem4/Subsystem2 ==
  u : Inport
  Integrator2 : Integrator
  Sqrt1 : Sqrt
  norm1 : MATLAB Function  TreatAsAtomicUnit=on
  Out1 : Outport
  wires:
  norm1/1(y) -> Integrator2/1
  Sqrt1/1 -> Out1/1
  Integrator2/1 -> Sqrt1/1
  u/1 -> norm1/1(u)

== system simulation_Hippocampus_compare_paper/Proposed Linear gain/HippCampus/Subsystem4/Subsystem3 ==
  u : Inport
  Integrator2 : Integrator
  Sqrt1 : Sqrt
  norm1 : MATLAB Function  TreatAsAtomicUnit=on
  Out1 : Outport
  wires:
  norm1/1(y) -> Integrator2/1
  Sqrt1/1 -> Out1/1
  Integrator2/1 -> Sqrt1/1
  u/1 -> norm1/1(u)

== system simulation_Hippocampus_compare_paper/Proposed Linear gain1/Disturbance: All derivatives1/disturbance3/Subsystem1 ==
  Clock : Clock
  Mux1 : Mux  Inputs=3
  wave frenquency : Subsystem
  wave percentage : Subsystem
  Out1 : Outport
  wires:
  wave frenquency/1(Out1) -> Mux1/2
  Mux1/1 -> Out1/1
  wave percentage/1(Out1) -> Mux1/1
  Clock/1 -> Mux1/3

== system simulation_Hippocampus_compare_paper/Proposed Linear gain1/HippCampus/Subsystem4/Subsystem ==
  u : Inport
  Integrator2 : Integrator
  Sqrt1 : Sqrt
  norm1 : MATLAB Function  TreatAsAtomicUnit=on
  Out1 : Outport
  wires:
  norm1/1(y) -> Integrator2/1
  Sqrt1/1 -> Out1/1
  Integrator2/1 -> Sqrt1/1
  u/1 -> norm1/1(u)

== system simulation_Hippocampus_compare_paper/Proposed Linear gain1/HippCampus/Subsystem4/Subsystem1 ==
  u : Inport
  Integrator2 : Integrator
  Sqrt1 : Sqrt
  norm1 : MATLAB Function  TreatAsAtomicUnit=on
  Out1 : Outport
  wires:
  norm1/1(y) -> Integrator2/1
  Sqrt1/1 -> Out1/1
  Integrator2/1 -> Sqrt1/1
  u/1 -> norm1/1(u)

== system simulation_Hippocampus_compare_paper/Proposed Linear gain1/HippCampus/Subsystem4/Subsystem2 ==
  u : Inport
  Integrator2 : Integrator
  Sqrt1 : Sqrt
  norm1 : MATLAB Function  TreatAsAtomicUnit=on
  Out1 : Outport
  wires:
  norm1/1(y) -> Integrator2/1
  Sqrt1/1 -> Out1/1
  Integrator2/1 -> Sqrt1/1
  u/1 -> norm1/1(u)

== system simulation_Hippocampus_compare_paper/Proposed Linear gain1/HippCampus/Subsystem4/Subsystem3 ==
  u : Inport
  Integrator2 : Integrator
  Sqrt1 : Sqrt
  norm1 : MATLAB Function  TreatAsAtomicUnit=on
  Out1 : Outport
  wires:
  norm1/1(y) -> Integrator2/1
  Sqrt1/1 -> Out1/1
  Integrator2/1 -> Sqrt1/1
  u/1 -> norm1/1(u)

== system simulation_Hippocampus_compare_paper/Proposed nonlinear gain/Disturbance: All derivatives1/disturbance3/Subsystem1 ==
  Clock : Clock
  Mux1 : Mux  Inputs=3
  wave frenquency : Subsystem
  wave percentage : Subsystem
  Out1 : Outport
  wires:
  wave frenquency/1(Out1) -> Mux1/2
  Mux1/1 -> Out1/1
  wave percentage/1(Out1) -> Mux1/1
  Clock/1 -> Mux1/3

== system simulation_Hippocampus_compare_paper/Proposed nonlinear gain/HippCampus/Subsystem4/Subsystem ==
  u : Inport
  Integrator2 : Integrator
  Sqrt1 : Sqrt
  norm1 : MATLAB Function  TreatAsAtomicUnit=on
  Out1 : Outport
  wires:
  norm1/1(y) -> Integrator2/1
  Sqrt1/1 -> Out1/1
  Integrator2/1 -> Sqrt1/1
  u/1 -> norm1/1(u)

== system simulation_Hippocampus_compare_paper/Proposed nonlinear gain/HippCampus/Subsystem4/Subsystem1 ==
  u : Inport
  Integrator2 : Integrator
  Sqrt1 : Sqrt
  norm1 : MATLAB Function  TreatAsAtomicUnit=on
  Out1 : Outport
  wires:
  norm1/1(y) -> Integrator2/1
  Sqrt1/1 -> Out1/1
  Integrator2/1 -> Sqrt1/1
  u/1 -> norm1/1(u)

== system simulation_Hippocampus_compare_paper/Proposed nonlinear gain/HippCampus/Subsystem4/Subsystem2 ==
  u : Inport
  Integrator2 : Integrator
  Sqrt1 : Sqrt
  norm1 : MATLAB Function  TreatAsAtomicUnit=on
  Out1 : Outport
  wires:
  norm1/1(y) -> Integrator2/1
  Sqrt1/1 -> Out1/1
  Integrator2/1 -> Sqrt1/1
  u/1 -> norm1/1(u)

== system simulation_Hippocampus_compare_paper/Proposed nonlinear gain/HippCampus/Subsystem4/Subsystem3 ==
  u : Inport
  Integrator2 : Integrator
  Sqrt1 : Sqrt
  norm1 : MATLAB Function  TreatAsAtomicUnit=on
  Out1 : Outport
  wires:
  norm1/1(y) -> Integrator2/1
  Sqrt1/1 -> Out1/1
  Integrator2/1 -> Sqrt1/1
  u/1 -> norm1/1(u)

== system simulation_Hippocampus_compare_paper/Proposed nonlinear gain1/Disturbance: All derivatives1/disturbance3/Subsystem1 ==
  Clock : Clock
  Mux1 : Mux  Inputs=3
  wave frenquency : Subsystem
  wave percentage : Subsystem
  Out1 : Outport
  wires:
  wave frenquency/1(Out1) -> Mux1/2
  Mux1/1 -> Out1/1
  wave percentage/1(Out1) -> Mux1/1
  Clock/1 -> Mux1/3

== system simulation_Hippocampus_compare_paper/Proposed nonlinear gain1/HippCampus/Subsystem4/Subsystem ==
  u : Inport
  Integrator2 : Integrator
  Sqrt1 : Sqrt
  norm1 : MATLAB Function  TreatAsAtomicUnit=on
  Out1 : Outport
  wires:
  norm1/1(y) -> Integrator2/1
  Sqrt1/1 -> Out1/1
  Integrator2/1 -> Sqrt1/1
  u/1 -> norm1/1(u)

== system simulation_Hippocampus_compare_paper/Proposed nonlinear gain1/HippCampus/Subsystem4/Subsystem1 ==
  u : Inport
  Integrator2 : Integrator
  Sqrt1 : Sqrt
  norm1 : MATLAB Function  TreatAsAtomicUnit=on
  Out1 : Outport
  wires:
  norm1/1(y) -> Integrator2/1
  Sqrt1/1 -> Out1/1
  Integrator2/1 -> Sqrt1/1
  u/1 -> norm1/1(u)

== system simulation_Hippocampus_compare_paper/Proposed nonlinear gain1/HippCampus/Subsystem4/Subsystem2 ==
  u : Inport
  Integrator2 : Integrator
  Sqrt1 : Sqrt
  norm1 : MATLAB Function  TreatAsAtomicUnit=on
  Out1 : Outport
  wires:
  norm1/1(y) -> Integrator2/1
  Sqrt1/1 -> Out1/1
  Integrator2/1 -> Sqrt1/1
  u/1 -> norm1/1(u)

== system simulation_Hippocampus_compare_paper/Proposed nonlinear gain1/HippCampus/Subsystem4/Subsystem3 ==
  u : Inport
  Integrator2 : Integrator
  Sqrt1 : Sqrt
  norm1 : MATLAB Function  TreatAsAtomicUnit=on
  Out1 : Outport
  wires:
  norm1/1(y) -> Integrator2/1
  Sqrt1/1 -> Out1/1
  Integrator2/1 -> Sqrt1/1
  u/1 -> norm1/1(u)

== system simulation_Hippocampus_compare_paper/Proposed nonlinear gain2/HippCampus/Subsystem4/Subsystem ==
  u : Inport
  Integrator2 : Integrator
  Sqrt1 : Sqrt
  norm1 : MATLAB Function  TreatAsAtomicUnit=on
  Out1 : Outport
  wires:
  norm1/1(y) -> Integrator2/1
  Sqrt1/1 -> Out1/1
  Integrator2/1 -> Sqrt1/1
  u/1 -> norm1/1(u)

== system simulation_Hippocampus_compare_paper/Proposed nonlinear gain2/HippCampus/Subsystem4/Subsystem1 ==
  u : Inport
  Integrator2 : Integrator
  Sqrt1 : Sqrt
  norm1 : MATLAB Function  TreatAsAtomicUnit=on
  Out1 : Outport
  wires:
  norm1/1(y) -> Integrator2/1
  Sqrt1/1 -> Out1/1
  Integrator2/1 -> Sqrt1/1
  u/1 -> norm1/1(u)

== system simulation_Hippocampus_compare_paper/Proposed nonlinear gain2/HippCampus/Subsystem4/Subsystem2 ==
  u : Inport
  Integrator2 : Integrator
  Sqrt1 : Sqrt
  norm1 : MATLAB Function  TreatAsAtomicUnit=on
  Out1 : Outport
  wires:
  norm1/1(y) -> Integrator2/1
  Sqrt1/1 -> Out1/1
  Integrator2/1 -> Sqrt1/1
  u/1 -> norm1/1(u)

== system simulation_Hippocampus_compare_paper/Proposed nonlinear gain2/HippCampus/Subsystem4/Subsystem3 ==
  u : Inport
  Integrator2 : Integrator
  Sqrt1 : Sqrt
  norm1 : MATLAB Function  TreatAsAtomicUnit=on
  Out1 : Outport
  wires:
  norm1/1(y) -> Integrator2/1
  Sqrt1/1 -> Out1/1
  Integrator2/1 -> Sqrt1/1
  u/1 -> norm1/1(u)

== system simulation_Hippocampus_compare_paper/Stabilizing without v w /HippCampus/Subsystem4/Subsystem ==
  u : Inport
  Integrator2 : Integrator
  Sqrt1 : Sqrt
  norm1 : MATLAB Function  TreatAsAtomicUnit=on
  Out1 : Outport
  wires:
  norm1/1(y) -> Integrator2/1
  Sqrt1/1 -> Out1/1
  Integrator2/1 -> Sqrt1/1
  u/1 -> norm1/1(u)

== system simulation_Hippocampus_compare_paper/Stabilizing without v w /HippCampus/Subsystem4/Subsystem1 ==
  u : Inport
  Integrator2 : Integrator
  Sqrt1 : Sqrt
  norm1 : MATLAB Function  TreatAsAtomicUnit=on
  Out1 : Outport
  wires:
  norm1/1(y) -> Integrator2/1
  Sqrt1/1 -> Out1/1
  Integrator2/1 -> Sqrt1/1
  u/1 -> norm1/1(u)

== system simulation_Hippocampus_compare_paper/Stabilizing without v w /HippCampus/Subsystem4/Subsystem2 ==
  u : Inport
  Integrator2 : Integrator
  Sqrt1 : Sqrt
  norm1 : MATLAB Function  TreatAsAtomicUnit=on
  Out1 : Outport
  wires:
  norm1/1(y) -> Integrator2/1
  Sqrt1/1 -> Out1/1
  Integrator2/1 -> Sqrt1/1
  u/1 -> norm1/1(u)

== system simulation_Hippocampus_compare_paper/Stabilizing without v w /HippCampus/Subsystem4/Subsystem3 ==
  u : Inport
  Integrator2 : Integrator
  Sqrt1 : Sqrt
  norm1 : MATLAB Function  TreatAsAtomicUnit=on
  Out1 : Outport
  wires:
  norm1/1(y) -> Integrator2/1
  Sqrt1/1 -> Out1/1
  Integrator2/1 -> Sqrt1/1
  u/1 -> norm1/1(u)

== system simulation_Hippocampus_compare_paper/Stabilizing without v w 1/HippCampus/Subsystem4/Subsystem ==
  u : Inport
  Integrator2 : Integrator
  Sqrt1 : Sqrt
  norm1 : MATLAB Function  TreatAsAtomicUnit=on
  Out1 : Outport
  wires:
  norm1/1(y) -> Integrator2/1
  Sqrt1/1 -> Out1/1
  Integrator2/1 -> Sqrt1/1
  u/1 -> norm1/1(u)

== system simulation_Hippocampus_compare_paper/Stabilizing without v w 1/HippCampus/Subsystem4/Subsystem1 ==
  u : Inport
  Integrator2 : Integrator
  Sqrt1 : Sqrt
  norm1 : MATLAB Function  TreatAsAtomicUnit=on
  Out1 : Outport
  wires:
  norm1/1(y) -> Integrator2/1
  Sqrt1/1 -> Out1/1
  Integrator2/1 -> Sqrt1/1
  u/1 -> norm1/1(u)

== system simulation_Hippocampus_compare_paper/Stabilizing without v w 1/HippCampus/Subsystem4/Subsystem2 ==
  u : Inport
  Integrator2 : Integrator
  Sqrt1 : Sqrt
  norm1 : MATLAB Function  TreatAsAtomicUnit=on
  Out1 : Outport
  wires:
  norm1/1(y) -> Integrator2/1
  Sqrt1/1 -> Out1/1
  Integrator2/1 -> Sqrt1/1
  u/1 -> norm1/1(u)

== system simulation_Hippocampus_compare_paper/Stabilizing without v w 1/HippCampus/Subsystem4/Subsystem3 ==
  u : Inport
  Integrator2 : Integrator
  Sqrt1 : Sqrt
  norm1 : MATLAB Function  TreatAsAtomicUnit=on
  Out1 : Outport
  wires:
  norm1/1(y) -> Integrator2/1
  Sqrt1/1 -> Out1/1
  Integrator2/1 -> Sqrt1/1
  u/1 -> norm1/1(u)

== system simulation_Hippocampus_compare_paper/NDI/Controller/Subsystem/Subsystem1/Subsystem ==
  x : Inport
  Demux : Demux  Outputs=12
  Mux : Mux  Inputs=3
  Terminator{,1..8} (9 alike) : Terminator
  rpy : Outport
  wires:
  x/1 -> Demux/1
  Demux/6 -> Mux/3
  Mux/1 -> rpy/1
  Demux/5 -> Mux/2
  Demux/4 -> Mux/1
  Demux/1 -> Terminator/1
  Demux/2 -> Terminator1/1
  Demux/3 -> Terminator2/1
  Demux/7 -> Terminator3/1
  Demux/9 -> Terminator5/1
  Demux/10 -> Terminator6/1
  Demux/11 -> Terminator7/1
  Demux/12 -> Terminator8/1
  Demux/8 -> Terminator4/1

== system simulation_Hippocampus_compare_paper/NDI/Controller/Subsystem/Subsystem2/NDI ==
  state : Inport
  Demux : Demux  Outputs=12
  Demux1 : Demux  Outputs=12
  Lf : MATLAB Function  TreatAsAtomicUnit=on
  Lg : MATLAB Function  TreatAsAtomicUnit=on
  Lg_h_inv : Outport
  Lf_h : Outport  Port=2
  wires:
  Demux/6 -> Lg/6(psi)
  Demux1/11 -> Lf/11(q)
  Demux/4 -> Lg/4(phi)
  Demux1/5 -> Lf/5(theta)
  Demux1/6 -> Lf/6(psi)
  Demux/2 -> Lg/2(y)
  Demux/7 -> Lg/7(u)
  Demux1/2 -> Lf/2(y)
  Demux1/1 -> Lf/1(x)
  state/1 -> Demux/1, Demux1/1
  Demux1/4 -> Lf/4(phi)
  Demux1/7 -> Lf/7(u)
  Demux/1 -> Lg/1(x)
  Demux/12 -> Lg/12(r)
  Demux/5 -> Lg/5(theta)
  Demux/8 -> Lg/8(v)
  Lf/1(Lf_h) -> Lf_h/1
  Demux/3 -> Lg/3(z)
  Demux/11 -> Lg/11(q)
  Demux1/8 -> Lf/8(v)
  Demux1/3 -> Lf/3(z)
  Demux/10 -> Lg/10(p)
  Demux1/12 -> Lf/12(r)
  Lg/1(Lg_h_inv) -> Lg_h_inv/1
  Demux1/9 -> Lf/9(w)
  Demux1/10 -> Lf/10(p)
  Demux/9 -> Lg/9(w)

== system simulation_Hippocampus_compare_paper/NDI/Controller/Subsystem/Subsystem2/Subsystem ==
  x : Inport
  Demux : Demux  Outputs=12
  Mux : Mux
  Terminator{1..8} (8 alike) : Terminator
  upqr : Outport
  wires:
  x/1 -> Demux/1
  Mux/1 -> upqr/1
  Demux/12 -> Mux/4
  Demux/11 -> Mux/3
  Demux/10 -> Mux/2
  Demux/7 -> Mux/1
  Demux/1 -> Terminator4/1
  Demux/2 -> Terminator1/1
  Demux/3 -> Terminator2/1
  Demux/4 -> Terminator3/1
  Demux/5 -> Terminator5/1
  Demux/6 -> Terminator6/1
  Demux/8 -> Terminator7/1
  Demux/9 -> Terminator8/1

== system simulation_Hippocampus_compare_paper/NDI/Disturbance: All derivatives1/disturbance3/Subsystem1/wave frenquency ==
  Constant2 : Constant
  Constant3 : Constant  Value=1.1
  Constant4 : Constant  Value=1.2
  Constant5 : Constant  Value=0.5
  Constant6 : Constant  Value=0.6
  Constant7 : Constant  Value=0.7
  Mux : Mux  Inputs=6
  Out1 : Outport
  wires:
  Constant3/1 -> Mux/2
  Constant2/1 -> Mux/1
  Constant4/1 -> Mux/3
  Constant7/1 -> Mux/6
  Mux/1 -> Out1/1
  Constant5/1 -> Mux/4
  Constant6/1 -> Mux/5

== system simulation_Hippocampus_compare_paper/NDI/Disturbance: All derivatives1/disturbance3/Subsystem1/wave percentage ==
  Constant{2..7} (6 alike) : Constant  Value=0
  Mux : Mux  Inputs=6
  Out1 : Outport
  wires:
  Constant3/1 -> Mux/2
  Constant2/1 -> Mux/1
  Constant4/1 -> Mux/3
  Constant7/1 -> Mux/6
  Mux/1 -> Out1/1
  Constant5/1 -> Mux/4
  Constant6/1 -> Mux/5

== system simulation_Hippocampus_compare_paper/NDI/Disturbance: All derivatives2/disturbance3/Subsystem1/wave frenquency ==
  Constant2 : Constant
  Constant3 : Constant  Value=1.1
  Constant4 : Constant  Value=1.2
  Constant5 : Constant  Value=0.5
  Constant6 : Constant  Value=0.6
  Constant7 : Constant  Value=0.7
  Mux : Mux  Inputs=6
  Out1 : Outport
  wires:
  Constant3/1 -> Mux/2
  Constant2/1 -> Mux/1
  Constant4/1 -> Mux/3
  Constant7/1 -> Mux/6
  Mux/1 -> Out1/1
  Constant5/1 -> Mux/4
  Constant6/1 -> Mux/5

== system simulation_Hippocampus_compare_paper/NDI/Disturbance: All derivatives2/disturbance3/Subsystem1/wave percentage ==
  Constant{2..7} (6 alike) : Constant  Value=0
  Mux : Mux  Inputs=6
  Out1 : Outport
  wires:
  Constant3/1 -> Mux/2
  Constant2/1 -> Mux/1
  Constant4/1 -> Mux/3
  Constant7/1 -> Mux/6
  Mux/1 -> Out1/1
  Constant5/1 -> Mux/4
  Constant6/1 -> Mux/5

== system simulation_Hippocampus_compare_paper/NDI4/Controller/Subsystem/Subsystem1/Subsystem ==
  x : Inport
  Demux : Demux  Outputs=12
  Mux : Mux  Inputs=3
  Terminator{,1..8} (9 alike) : Terminator
  rpy : Outport
  wires:
  x/1 -> Demux/1
  Demux/6 -> Mux/3
  Mux/1 -> rpy/1
  Demux/5 -> Mux/2
  Demux/4 -> Mux/1
  Demux/1 -> Terminator/1
  Demux/2 -> Terminator1/1
  Demux/3 -> Terminator2/1
  Demux/7 -> Terminator3/1
  Demux/9 -> Terminator5/1
  Demux/10 -> Terminator6/1
  Demux/11 -> Terminator7/1
  Demux/12 -> Terminator8/1
  Demux/8 -> Terminator4/1

== system simulation_Hippocampus_compare_paper/NDI4/Controller/Subsystem/Subsystem2/NDI ==
  state : Inport
  Demux : Demux  Outputs=12
  Demux1 : Demux  Outputs=12
  Lf : MATLAB Function  TreatAsAtomicUnit=on
  Lg : MATLAB Function  TreatAsAtomicUnit=on
  Lg_h_inv : Outport
  Lf_h : Outport  Port=2
  wires:
  Demux/6 -> Lg/6(psi)
  Demux1/11 -> Lf/11(q)
  Demux/4 -> Lg/4(phi)
  Demux1/5 -> Lf/5(theta)
  Demux1/6 -> Lf/6(psi)
  Demux/2 -> Lg/2(y)
  Demux/7 -> Lg/7(u)
  Demux1/2 -> Lf/2(y)
  Demux1/1 -> Lf/1(x)
  state/1 -> Demux/1, Demux1/1
  Demux1/4 -> Lf/4(phi)
  Demux1/7 -> Lf/7(u)
  Demux/1 -> Lg/1(x)
  Demux/12 -> Lg/12(r)
  Demux/5 -> Lg/5(theta)
  Demux/8 -> Lg/8(v)
  Lf/1(Lf_h) -> Lf_h/1
  Demux/3 -> Lg/3(z)
  Demux/11 -> Lg/11(q)
  Demux1/8 -> Lf/8(v)
  Demux1/3 -> Lf/3(z)
  Demux/10 -> Lg/10(p)
  Demux1/12 -> Lf/12(r)
  Lg/1(Lg_h_inv) -> Lg_h_inv/1
  Demux1/9 -> Lf/9(w)
  Demux1/10 -> Lf/10(p)
  Demux/9 -> Lg/9(w)

== system simulation_Hippocampus_compare_paper/NDI4/Controller/Subsystem/Subsystem2/Subsystem ==
  x : Inport
  Demux : Demux  Outputs=12
  Mux : Mux
  Terminator{1..8} (8 alike) : Terminator
  upqr : Outport
  wires:
  x/1 -> Demux/1
  Mux/1 -> upqr/1
  Demux/12 -> Mux/4
  Demux/11 -> Mux/3
  Demux/10 -> Mux/2
  Demux/7 -> Mux/1
  Demux/1 -> Terminator4/1
  Demux/2 -> Terminator1/1
  Demux/3 -> Terminator2/1
  Demux/4 -> Terminator3/1
  Demux/5 -> Terminator5/1
  Demux/6 -> Terminator6/1
  Demux/8 -> Terminator7/1
  Demux/9 -> Terminator8/1

== system simulation_Hippocampus_compare_paper/NDI4/Disturbance: All derivatives1/disturbance3/Subsystem1/wave frenquency ==
  Constant2 : Constant
  Constant3 : Constant  Value=1.1
  Constant4 : Constant  Value=1.2
  Constant5 : Constant  Value=0.5
  Constant6 : Constant  Value=0.6
  Constant7 : Constant  Value=0.7
  Mux : Mux  Inputs=6
  Out1 : Outport
  wires:
  Constant3/1 -> Mux/2
  Constant2/1 -> Mux/1
  Constant4/1 -> Mux/3
  Constant7/1 -> Mux/6
  Mux/1 -> Out1/1
  Constant5/1 -> Mux/4
  Constant6/1 -> Mux/5

== system simulation_Hippocampus_compare_paper/NDI4/Disturbance: All derivatives1/disturbance3/Subsystem1/wave percentage ==
  Constant{2..7} (6 alike) : Constant  Value=0
  Mux : Mux  Inputs=6
  Out1 : Outport
  wires:
  Constant3/1 -> Mux/2
  Constant2/1 -> Mux/1
  Constant4/1 -> Mux/3
  Constant7/1 -> Mux/6
  Mux/1 -> Out1/1
  Constant5/1 -> Mux/4
  Constant6/1 -> Mux/5
